simulink library "CanadianSolar"  (R2017a)
settings: Solver=VariableStepAuto  StartTime=0.0  StopTime=10.0  RelTol=1e-3
libraries: elec_lib x60
settings Model: Creator=Nikhil Kilari  LastModifiedBy=Nikhil Kilari

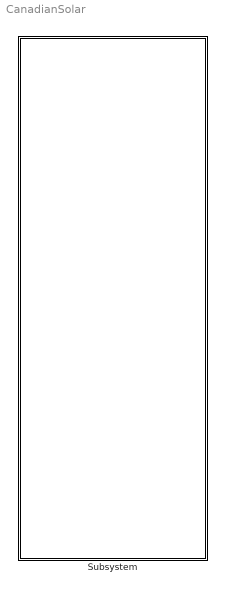
== system CanadianSolar ==
  Subsystem : Subsystem

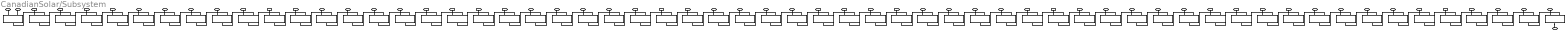
== system CanadianSolar/Subsystem ==
  Sol{1..60} (60 alike) : elec_lib/Sources/Solar Cell  prm=1  Isc=8.87 A  Voc=0.66166667 V  Is=1e-6 A  Is2=0 A  Iph=7.34 A  Ir0=1000 W/m^2  ec=1.0506  N2=2  Rs=0.00572567 Ohm  Rp=Inf Ohm  N_series=1  TIPH1=0 1/K  EG=1.11 eV  TXIS1=3  TXIS2=3  TRS1=0  TRP1=0  Tmeas=25 degC  TFIXED=25 degC  thermal_mass=100 J/K  initial_temperature=25 degC
      settings: SourceProductName=Simscape Electronics  SourceProductBaseCode=SN
  Conn1 : PMIOPort  Port=1  Side=Left
  Conn2 : PMIOPort  Port=2  Side=Left
  Conn3 : PMIOPort  Port=3  Side=Left
  Conn4 : PMIOPort  Port=4  Side=Left
  Conn5 : PMIOPort  Port=5  Side=Left
  Conn6 : PMIOPort  Port=6  Side=Left
  Conn7 : PMIOPort  Port=7  Side=Left
  Conn8 : PMIOPort  Port=8  Side=Left
  Conn9 : PMIOPort  Port=9  Side=Left
  Conn10 : PMIOPort  Port=10  Side=Left
  Conn11 : PMIOPort  Port=11  Side=Left
  Conn12 : PMIOPort  Port=12  Side=Left
  Conn13 : PMIOPort  Port=13  Side=Left
  Conn14 : PMIOPort  Port=14  Side=Left
  Conn15 : PMIOPort  Port=15  Side=Left
  Conn16 : PMIOPort  Port=16  Side=Left
  Conn17 : PMIOPort  Port=17  Side=Left
  Conn18 : PMIOPort  Port=18  Side=Left
  Conn19 : PMIOPort  Port=19  Side=Left
  Conn20 : PMIOPort  Port=20  Side=Left
  Conn21 : PMIOPort  Port=21  Side=Left
  Conn22 : PMIOPort  Port=22  Side=Left
  Conn23 : PMIOPort  Port=23  Side=Left
  Conn24 : PMIOPort  Port=24  Side=Left
  Conn25 : PMIOPort  Port=25  Side=Left
  Conn26 : PMIOPort  Port=26  Side=Left
  Conn27 : PMIOPort  Port=27  Side=Left
  Conn28 : PMIOPort  Port=28  Side=Left
  Conn29 : PMIOPort  Port=29  Side=Left
  Conn30 : PMIOPort  Port=30  Side=Left
  Conn31 : PMIOPort  Port=31  Side=Left
  Conn32 : PMIOPort  Port=32  Side=Left
  Conn33 : PMIOPort  Port=33  Side=Left
  Conn34 : PMIOPort  Port=34  Side=Left
  Conn35 : PMIOPort  Port=35  Side=Left
  Conn36 : PMIOPort  Port=36  Side=Left
  Conn37 : PMIOPort  Port=37  Side=Left
  Conn38 : PMIOPort  Port=38  Side=Left
  Conn39 : PMIOPort  Port=39  Side=Left
  Conn40 : PMIOPort  Port=40  Side=Left
  Conn41 : PMIOPort  Port=41  Side=Left
  Conn42 : PMIOPort  Port=42  Side=Left
  Conn43 : PMIOPort  Port=43  Side=Left
  Conn44 : PMIOPort  Port=44  Side=Left
  Conn45 : PMIOPort  Port=45  Side=Left
  Conn46 : PMIOPort  Port=46  Side=Left
  Conn47 : PMIOPort  Port=47  Side=Left
  Conn48 : PMIOPort  Port=48  Side=Left
  Conn49 : PMIOPort  Port=49  Side=Left
  Conn50 : PMIOPort  Port=50  Side=Left
  Conn51 : PMIOPort  Port=51  Side=Left
  Conn52 : PMIOPort  Port=52  Side=Left
  Conn53 : PMIOPort  Port=53  Side=Left
  Conn54 : PMIOPort  Port=54  Side=Left
  Conn55 : PMIOPort  Port=55  Side=Left
  Conn56 : PMIOPort  Port=56  Side=Left
  Conn57 : PMIOPort  Port=57  Side=Left
  Conn58 : PMIOPort  Port=58  Side=Left
  Conn59 : PMIOPort  Port=59  Side=Left
  Conn60 : PMIOPort  Port=60  Side=Left
  Conn61 : PMIOPort  Port=61  Side=Left
  Conn62 : PMIOPort  Port=62  Side=Right
  connections:
  Sol54/LConn1 -- Conn55/RConn1
  Sol52/LConn1 -- Conn53/RConn1
  Sol15/LConn1 -- Conn16/RConn1
  Sol18/LConn1 -- Conn19/RConn1
  Sol13/LConn1 -- Conn14/RConn1
  Sol1/LConn1 -- Conn1/RConn1
  Sol1/LConn2 -- Conn2/RConn1
  Sol17/LConn1 -- Conn18/RConn1
  Sol15/LConn2 -- Sol14/RConn1
  Sol23/LConn2 -- Sol22/RConn1
  Sol37/LConn2 -- Sol36/RConn1
  Sol45/LConn2 -- Sol44/RConn1
  Sol2/LConn2 -- Sol1/RConn1
  Sol50/LConn2 -- Sol49/RConn1
  Sol54/LConn2 -- Sol53/RConn1
  Sol52/LConn2 -- Sol51/RConn1
  Sol59/LConn2 -- Sol58/RConn1
  Sol43/LConn1 -- Conn44/RConn1
  Sol11/LConn1 -- Conn12/RConn1
  Sol7/LConn1 -- Conn8/RConn1
  Sol35/LConn1 -- Conn36/RConn1
  Sol41/LConn1 -- Conn42/RConn1
  Sol33/LConn1 -- Conn34/RConn1
  Sol9/LConn1 -- Conn10/RConn1
  Sol38/LConn1 -- Conn39/RConn1
  Sol4/LConn1 -- Conn5/RConn1
  Sol20/LConn1 -- Conn21/RConn1
  Sol28/LConn1 -- Conn29/RConn1
  Sol19/LConn1 -- Conn20/RConn1
  Sol21/LConn1 -- Conn22/RConn1
  Sol51/LConn1 -- Conn52/RConn1
  Sol10/LConn1 -- Conn11/RConn1
  Sol27/LConn1 -- Conn28/RConn1
  Sol37/LConn1 -- Conn38/RConn1
  Sol34/LConn1 -- Conn35/RConn1
  Sol46/LConn1 -- Conn47/RConn1
  Sol31/LConn1 -- Conn32/RConn1
  Sol3/LConn1 -- Conn4/RConn1
  Sol44/LConn1 -- Conn45/RConn1
  Sol5/LConn1 -- Conn6/RConn1
  Sol8/LConn1 -- Conn9/RConn1
  Sol12/LConn2 -- Sol11/RConn1
  Sol24/LConn1 -- Conn25/RConn1
  Sol24/LConn2 -- Sol23/RConn1
  Sol29/LConn2 -- Sol28/RConn1
  Sol36/LConn2 -- Sol35/RConn1
  Sol25/LConn1 -- Conn26/RConn1
  Sol33/LConn2 -- Sol32/RConn1
  Sol40/LConn2 -- Sol39/RConn1
  Sol39/LConn2 -- Sol38/RConn1
  Sol48/LConn2 -- Sol47/RConn1
  Sol47/LConn2 -- Sol46/RConn1
  Sol58/LConn2 -- Sol57/RConn1
  Sol55/LConn2 -- Sol54/RConn1
  Sol57/LConn2 -- Sol56/RConn1
  Sol56/LConn2 -- Sol55/RConn1
  Sol16/LConn1 -- Conn17/RConn1
  Sol60/LConn1 -- Conn61/RConn1
  Sol32/LConn1 -- Conn33/RConn1
  Sol58/LConn1 -- Conn59/RConn1
  Sol36/LConn1 -- Conn37/RConn1
  Sol39/LConn1 -- Conn40/RConn1
  Sol57/LConn1 -- Conn58/RConn1
  Sol22/LConn1 -- Conn23/RConn1
  Sol60/RConn1 -- Conn62/RConn1
  Sol29/LConn1 -- Conn30/RConn1
  Sol2/LConn1 -- Conn3/RConn1
  Sol40/LConn1 -- Conn41/RConn1
  Sol55/LConn1 -- Conn56/RConn1
  Sol48/LConn1 -- Conn49/RConn1
  Sol26/LConn1 -- Conn27/RConn1
  Sol53/LConn1 -- Conn54/RConn1
  Sol49/LConn1 -- Conn50/RConn1
  Sol47/LConn1 -- Conn48/RConn1
  Sol6/LConn1 -- Conn7/RConn1
  Sol42/LConn1 -- Conn43/RConn1
  Sol56/LConn1 -- Conn57/RConn1
  Sol59/LConn1 -- Conn60/RConn1
  Sol30/LConn1 -- Conn31/RConn1
  Sol45/LConn1 -- Conn46/RConn1
  Sol4/LConn2 -- Sol3/RConn1
  Sol50/LConn1 -- Conn51/RConn1
  Sol14/LConn2 -- Sol13/RConn1
  Sol13/LConn2 -- Sol12/RConn1
  Sol12/LConn1 -- Conn13/RConn1
  Sol17/LConn2 -- Sol16/RConn1
  Sol14/LConn1 -- Conn15/RConn1
  Sol23/LConn1 -- Conn24/RConn1
  Sol44/LConn2 -- Sol43/RConn1
  Sol42/LConn2 -- Sol41/RConn1
  Sol43/LConn2 -- Sol42/RConn1
  Sol49/LConn2 -- Sol48/RConn1
  Sol3/LConn2 -- Sol2/RConn1
  Sol7/LConn2 -- Sol6/RConn1
  Sol9/LConn2 -- Sol8/RConn1
  Sol8/LConn2 -- Sol7/RConn1
  Sol10/LConn2 -- Sol9/RConn1
  Sol11/LConn2 -- Sol10/RConn1
  Sol19/LConn2 -- Sol18/RConn1
  Sol18/LConn2 -- Sol17/RConn1
  Sol21/LConn2 -- Sol20/RConn1
  Sol22/LConn2 -- Sol21/RConn1
  Sol25/LConn2 -- Sol24/RConn1
  Sol31/LConn2 -- Sol30/RConn1
  Sol30/LConn2 -- Sol29/RConn1
  Sol35/LConn2 -- Sol34/RConn1
  Sol34/LConn2 -- Sol33/RConn1
  Sol38/LConn2 -- Sol37/RConn1
  Sol41/LConn2 -- Sol40/RConn1
  Sol46/LConn2 -- Sol45/RConn1
  Sol53/LConn2 -- Sol52/RConn1
  Sol51/LConn2 -- Sol50/RConn1
  Sol60/LConn2 -- Sol59/RConn1
  Sol6/LConn2 -- Sol5/RConn1
  Sol5/LConn2 -- Sol4/RConn1
  Sol16/LConn2 -- Sol15/RConn1
  Sol20/LConn2 -- Sol19/RConn1
  Sol27/LConn2 -- Sol26/RConn1
  Sol28/LConn2 -- Sol27/RConn1
  Sol26/LConn2 -- Sol25/RConn1
  Sol32/LConn2 -- Sol31/RConn1
